simulink model "xTyTbeta1beta2"  (Simulink 7.2)
settings: Solver=FixedStepDiscrete  StartTime=0.0  StopTime=TF  FixedStep=5e-2  RelTol=1e-4
values from neighbouring files (symbols this model uses):
  Lb1 = 0.3    [gns_robot_planare.m]    (also in s_robot_planare.m)
  Lb2 = 0.4    [gns_robot_planare.m]    (also in s_robot_planare.m)
settings Model: Creator=prof. G. Celentano  LastModifiedBy=gle
settings OptimizationCC: InitFltsAndDblsToZero=on
settings DebuggingCC: SaveWithParameterizedLinksMsg=none
settings GRTTargetCC: TargetFcnLib=ansi_tfl_tmw.mat

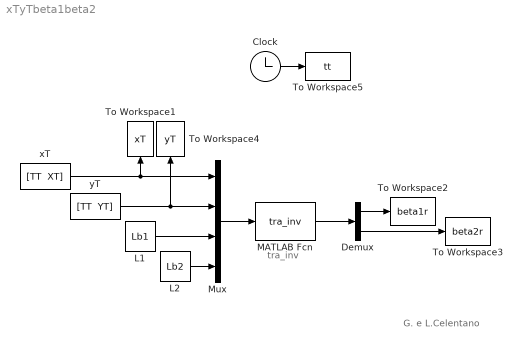
== system xTyTbeta1beta2 ==
  note: tra_inv
  note: G. e L.Celentano
  Clock : Clock
      settings: Decimation=10
  Demux : Demux  Outputs=2
  L1 : Constant  Value=Lb1  OutDataType=sfix(16)  OutScaling=2^0
  L2 : Constant  Value=Lb2  OutDataType=sfix(16)  OutScaling=2^0
  MATLAB Fcn : MATLABFcn  MATLABFcn=tra_inv
  Mux : Mux
  To Workspace1 : ToWorkspace  VariableName=xT  SampleTime=-1  SaveFormat=Array
      settings: Orientation=up
  To Workspace2 : ToWorkspace  VariableName=beta1r  SampleTime=-1  SaveFormat=Array
  To Workspace3 : ToWorkspace  VariableName=beta2r  SampleTime=-1  SaveFormat=Array
  To Workspace4 : ToWorkspace  VariableName=yT  SampleTime=-1  SaveFormat=Array
      settings: Orientation=up
  To Workspace5 : ToWorkspace  VariableName=tt  SampleTime=-1  SaveFormat=Array
  xT : FromWorkspace  VariableName="[TT  XT]"  SampleTime=0
  yT : FromWorkspace  VariableName="[TT  YT]"  SampleTime=0
  wires:
  Mux/1 -> MATLAB Fcn/1
  xT/1 -> Mux/1, To Workspace1/1
  yT/1 -> Mux/2, To Workspace4/1
  MATLAB Fcn/1 -> Demux/1
  Demux/1 -> To Workspace2/1
  Demux/2 -> To Workspace3/1
  L1/1 -> Mux/3
  L2/1 -> Mux/4
  Clock/1 -> To Workspace5/1
